simulink model "CurrentRelay"  (R2015b)
settings: Solver=FixedStepAuto  StartTime=0.0  StopTime=5  FixedStep=1e-5  RelTol=1e-3
libraries: powerlib x12
settings Model: Creator=yoush  LastModifiedBy=yoush

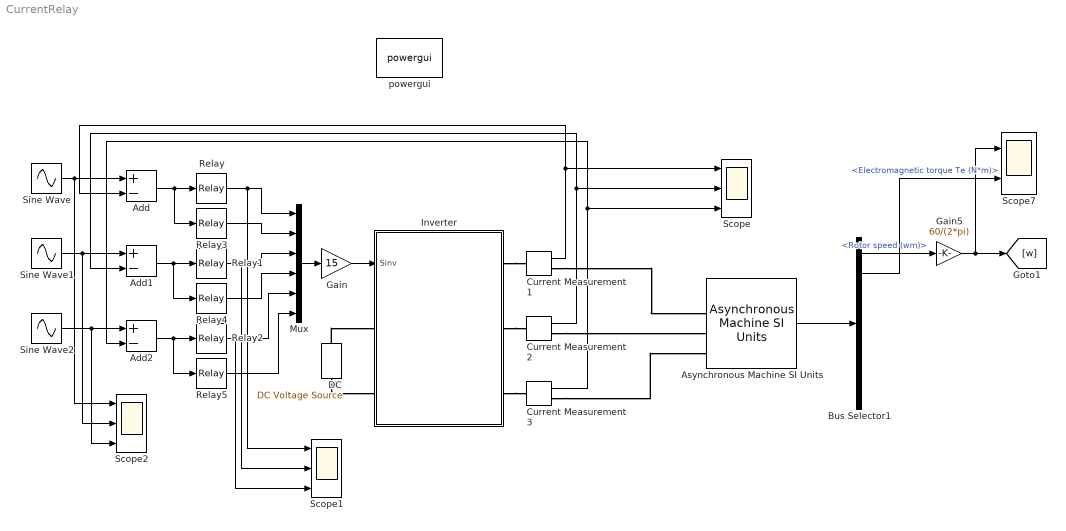
== system CurrentRelay ==
  Add : Sum  Inputs=+-
  Add1 : Sum  Inputs=+-
  Add2 : Sum  Inputs=+-
  Asynchronous Machine SI Units : powerlib/Machines/Asynchronous Machine SI Units  RotorType=Squirrel-cage  PresetModel=No  MechanicalLoad=Torque Tm  ShowDetailedParameters=on  ReferenceFrame=Stationary  Units=SI  MeasurementBus=off  NominalParameters=[22000 380 50]  Stator=[0.435 2e-3]  Rotor=[0.816 2e-3]  Cage1=[0.4155 0.002066]  Cage2=[0.4168 0.0003495]  Lm=69.31e-3  Mechanical=[0.089 0 2]  PolePairs=2  InitialConditions=[ 1 0 0 0 0 0 0 0]  SimulateSaturation=off  Saturation=[14.03593122, 27.81365428, 53.79336849, 72.68890987, 97.98006896, 148.6815601, 215.7428561, 302.9841135, 428.7778367 ; 230, 322, 414, 460, 506, 552, 598, 644, 690]  LoadFlowParameters=1492000  TsPowergui=0  TsBlock=-1  IterativeModel=Trapezoidal non iterative  Pmec=1.492e+006
  Bus Selector1 : BusSelector  OutputSignals="Mechanical.Rotor speed (wm),Mechanical.Electromagnetic torque Te (N*m),Stator measurements.Stator voltage vs_d (V),Stator measurements.Stator voltage vs_q (V),Stator measurements.Stator current is_d (A),Stator measurements.Stator current  is_q (A),Rotor measurements.Rotor flux phir_d (V s),Rotor measurements.Rotor flux phir_q (V s)"
  Current Measurement1 : powerlib/Measurements/Current Measurement  PhasorSimulation=off  OutputType=Complex  PSBequivalent=0
  Current Measurement2 : powerlib/Measurements/Current Measurement  PhasorSimulation=off  OutputType=Complex  PSBequivalent=0
  Current Measurement3 : powerlib/Measurements/Current Measurement  PhasorSimulation=off  OutputType=Complex  PSBequivalent=0
  DC : powerlib/Electrical Sources/DC Voltage Source  Amplitude=400  Measurements=None
  Gain : Gain  Gain=15
  Gain5 : Gain  Gain=60/(2*pi)
  Inverter : Subsystem
  Mux : Mux  Inputs=6
  Relay : Relay  OnSwitchValue=0.5  OffSwitchValue=-0.5
  Relay1 : Relay  OnSwitchValue=0.5  OffSwitchValue=-0.5
  Relay2 : Relay  OnSwitchValue=0.5  OffSwitchValue=-0.5
  Relay3 : Relay  OnSwitchValue=0.5  OffSwitchValue=-0.5  OnOutputValue=0  OffOutputValue=1
  Relay4 : Relay  OnSwitchValue=0.5  OffSwitchValue=-0.5  OnOutputValue=0  OffOutputValue=1
  Relay5 : Relay  OnSwitchValue=0.5  OffSwitchValue=-0.5  OnOutputValue=0  OffOutputValue=1
  Scope : Scope  NumInputPorts=3
  Scope1 : Scope  NumInputPorts=3
  Scope2 : Scope  NumInputPorts=3
  Scope7 : Scope  NumInputPorts=2
  Sine Wave : Sin  Amplitude=10  Frequency=100*pi  SampleTime=0
  Sine Wave1 : Sin  Amplitude=10  Frequency=100*pi  Phase=-2/3*pi  SampleTime=0
  Sine Wave2 : Sin  Amplitude=10  Frequency=100*pi  Phase=2/3*pi  SampleTime=0
  powergui : powerlib/powergui  Priority=1  SimulationMode=Continuous  SolverType=Tustin/Backward Euler (TBE)  SampleTime=1e-4  frequency=60  SPID=off  DisableSnubberDevices=off  DisableRonSwitches=off  DisableVfSwitches=off  SwTol=0  DisplayEquations=off  Interpol=off  ExternalGateDelay=off  methode=off  Ts=10  FunctionMessages=off  echomessages=off  HookPort=off  EnableUseOfTLC=off  x0status=blocks  frequencyindice=50  Pbase=100e6  ErrMax=1e-4  Iterations=50  UnitsV=kV  UnitsW=MW  buscounter=0  RestoreLinks=warning  ResistiveCurrentMeasurement=off  Frange=[0:2:500]  Ylog=off  Xlog=on  ShowGrid=off  save=off  variable=ZData  structure=we  ZoomFFT=off  StartTime=0.4  cycles=5  DisplayStyle=2  fundamental=100  FreqAxis=off  MaxFrequency=1000  frequencyindicesteady=1  RmsSteady=1  display=off
  wires:
  Sine Wave/1 -> Scope2/1, Add/1
  Add/1 -> Relay3/1, Relay/1
  Add1/1 -> Relay4/1, Relay1/1
  Add2/1 -> Relay5/1, Relay2/1
  Sine Wave2/1 -> Scope2/3, Add2/1
  Sine Wave1/1 -> Scope2/2, Add1/1
  Current Measurement1/1 -> Scope/1, Add/2
  Current Measurement2/1 -> Scope/2, Add1/2
  Current Measurement3/1 -> Scope/3, Add2/2
  Gain/1 -> Inverter/1(Sinv)
  Mux/1 -> Gain/1
  Relay/1 -> Scope1/1, Mux/1
  Relay3/1 -> Mux/2
  Relay1/1 -> Scope1/2, Mux/3
  Relay4/1 -> Mux/4
  Relay2/1 -> Scope1/3, Mux/5
  Relay5/1 -> Mux/6
  Asynchronous Machine SI Units/1 -> Bus Selector1/1
  Bus Selector1/1 -> Gain5/1  "<Rotor speed (wm)>"
  Gain5/1 -> Scope7/1, [w]
  Bus Selector1/2 -> Scope7/2  "<Electromagnetic torque Te (N*m)>"
  connections:
  Inverter/RConn1 -- Current Measurement1/LConn1
  Inverter/RConn2 -- Current Measurement2/LConn1
  Inverter/RConn3 -- Current Measurement3/LConn1
  Current Measurement1/RConn1 -- Asynchronous Machine SI Units/LConn1
  Current Measurement2/RConn1 -- Asynchronous Machine SI Units/LConn2
  Current Measurement3/RConn1 -- Asynchronous Machine SI Units/LConn3
  DC/RConn1 -- Inverter/LConn1
  DC/LConn1 -- Inverter/LConn2

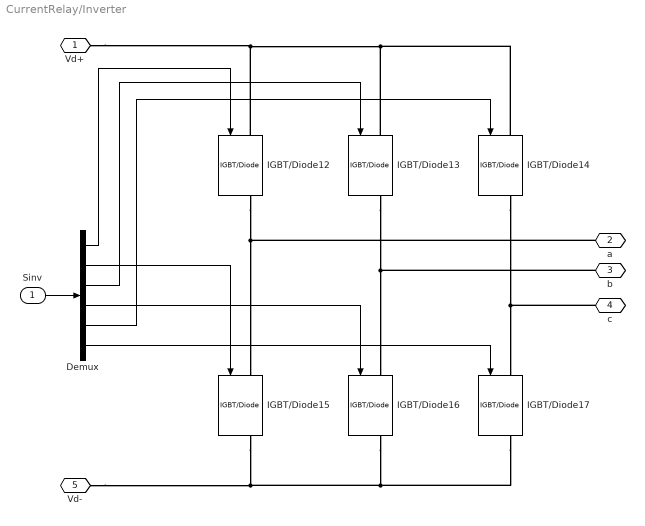
== system CurrentRelay/Inverter ==
  Sinv : Inport
  Demux : Demux  Outputs=6
  IGBT/Diode{12..17} (6 alike) : powerlib/Power Electronics/IGBT//Diode  Ron=1e-3  Rs=1e5  Cs=inf  Measurements=on
  Vd+ : PMIOPort  Port=1  Side=Left
  a : PMIOPort  Port=2  Side=Right
  b : PMIOPort  Port=3  Side=Right
  c : PMIOPort  Port=4  Side=Right
  Vd- : PMIOPort  Port=5  Side=Left
  wires:
  Demux/5 -> IGBT/Diode14/1
  Demux/4 -> IGBT/Diode16/1
  Demux/3 -> IGBT/Diode13/1
  Demux/6 -> IGBT/Diode17/1
  Demux/1 -> IGBT/Diode12/1
  Sinv/1 -> Demux/1
  Demux/2 -> IGBT/Diode15/1
  connections:
  IGBT/Diode12/RConn1 -- IGBT/Diode15/LConn1 -- a/RConn1
  IGBT/Diode13/RConn1 -- IGBT/Diode16/LConn1 -- b/RConn1
  IGBT/Diode14/RConn1 -- IGBT/Diode17/LConn1 -- c/RConn1
  IGBT/Diode17/RConn1 -- IGBT/Diode16/RConn1 -- Vd-/RConn1 -- IGBT/Diode15/RConn1
  IGBT/Diode12/LConn1 -- Vd+/RConn1 -- IGBT/Diode13/LConn1 -- IGBT/Diode14/LConn1
